simulink model "PEMFuelCellSystemWithACustomLibrary"  (R2025b)
settings: Solver=VariableStepAuto  StartTime=0.0  StopTime=2500  RelTol=1e-3  AbsTol=1e-3
model workspace: external: MATLAB File PEMFuelCellSystemWithACustomLibraryParameters.m (data not in the file)
values from neighbouring files (symbols this model uses):
  anode_tube_D = 0.01    [PEMFuelCellSystemWithACustomLibraryParameters.m]
  cathode_tube_D = 0.05    [PEMFuelCellSystemWithACustomLibraryParameters.m]
  comp_rpm_TLU = [0, 1800, 3600]    [PEMFuelCellSystemWithACustomLibraryParameters.m]
  coolant_num_layers = 20    [PEMFuelCellSystemWithACustomLibraryParameters.m]
  coolant_num_passes = 12    [PEMFuelCellSystemWithACustomLibraryParameters.m]
  coolant_tube_D = 0.05    [PEMFuelCellSystemWithACustomLibraryParameters.m]
  coolant_w_channels = 1    [PEMFuelCellSystemWithACustomLibraryParameters.m]
  env_p = 0.101325    [PEMFuelCellSystemWithACustomLibraryParameters.m]
  env_T = 20    [PEMFuelCellSystemWithACustomLibraryParameters.m]
  env_yH20 = env_RH * env_pSat_H2O / env_p    [PEMFuelCellSystemWithACustomLibraryParameters.m]
  env_yO2 = 0.21    [PEMFuelCellSystemWithACustomLibraryParameters.m]
  radiator_air_area_fins = 2 * radiator_N_fins * radiator_W * radiator_gap_H    (= 11.5625)    [PEMFuelCellSystemWithACustomLibraryParameters.m]
  radiator_air_area_primary = 2 * (radiator_N_tubes - 1) * radiator_W * (radiator_L + radiator_gap_H)    (= 1.223125)    [PEMFuelCellSystemWithACustomLibraryParameters.m]
  radiator_eta_fin = 0.7    [PEMFuelCellSystemWithACustomLibraryParameters.m]
  radiator_N_tubes = 25    [PEMFuelCellSystemWithACustomLibraryParameters.m]
  radiator_rho = 2700    [PEMFuelCellSystemWithACustomLibraryParameters.m]
  radiator_t_wall = 1e-4    (= 0.0001)    [PEMFuelCellSystemWithACustomLibraryParameters.m]
  radiator_tube_H = 0.0015    [PEMFuelCellSystemWithACustomLibraryParameters.m]
  radiator_W = 0.025    [PEMFuelCellSystemWithACustomLibraryParameters.m]
  stack_area = 280    [PEMFuelCellSystemWithACustomLibraryParameters.m]
  stack_iL = 1.4    [PEMFuelCellSystemWithACustomLibraryParameters.m]
  stack_mea_rho = 1800    [PEMFuelCellSystemWithACustomLibraryParameters.m]
  stack_num_cells = 400    [PEMFuelCellSystemWithACustomLibraryParameters.m]
  stack_num_channels = 8    [PEMFuelCellSystemWithACustomLibraryParameters.m]
  stack_t_gdl = 250    [PEMFuelCellSystemWithACustomLibraryParameters.m]
  stack_t_membrane = 125    [PEMFuelCellSystemWithACustomLibraryParameters.m]
  stack_w_channels = 1    [PEMFuelCellSystemWithACustomLibraryParameters.m]
libraries: fl_lib x57, FuelCell_lib x32, nesl_utility x24, slpidlib x2, simulink x1
(part 1 of 3)
CloseFcn:
  | try,close(h1_PEMFuelCellSystemWithACustomLibrary),end
  | clear h1_PEMFuelCellSystemWithACustomLibrary
  | try,close(h2_PEMFuelCellSystemWithACustomLibrary),end
  | clear h2_PEMFuelCellSystemWithACustomLibrary
  | try,close(h3_PEMFuelCellSystemWithACustomLibrary),end
  | clear h3_PEMFuelCellSystemWithACustomLibrary
  | try,close(h4_PEMFuelCellSystemWithACustomLibrary),end
  | clear h4_PEMFuelCellSystemWithACustomLibrary
  | try,close(h5_PEMFuelCellSystemWithACustomLibrary),end
  | clear h5_PEMFuelCellSystemWithACustomLibrary
  | try,close(h6_PEMFuelCellSystemWithACustomLibrary),end
  | clear h6_PEMFuelCellSystemWithACustomLibrary
  | 
  | clear tout simlog_PEMFuelCellSystemWithACustomLibrary
Description:
  | PEM Fuel Cell System with a Custom Library
settings Model: Creator=The MathWorks, Inc.  LastModifiedBy=The MathWorks, Inc.
settings SolverCC: AutoScaleAbsTol=off  MaxConsecutiveMinStep=10  AlgebraicLoopSolver=TrustRegion  MaxZcPerStep=1.0
settings DataIOCC: SaveFormat=Array  ReturnWorkspaceOutputs=off
settings DebuggingCC: UnconnectedInputMsg=warning  UnconnectedOutputMsg=warning  UnconnectedLineMsg=warning  SymbolicDimsDataTypeCodeGenerationDiagnostic=none
settings ModelReferenceCC: EnableRefExpFcnMdlSchedulingChecks=on
settings SFSimCC: CustomCodeUndefinedFunction=UseInterfaceOnly
settings RTWCC: GPUComputeCapability=3.5  DLArmComputeVersion=19.05
settings SimscapeCC: SimscapeLogType=all  SimscapeLogSimulationStatistics=on  SimscapeLogName=simlog_PEMFuelCellSystemWithACustomLibrary  SimscapeLogDataHistory=20000.0

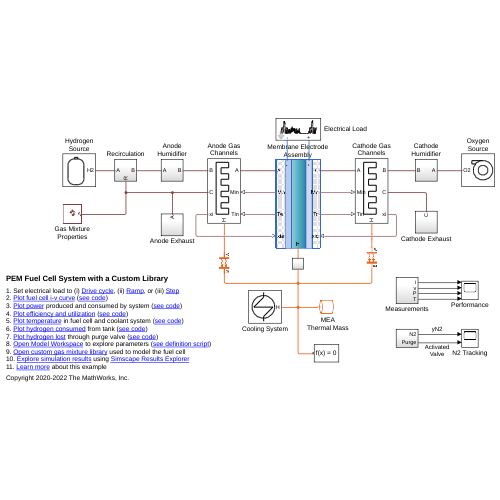
[thumbnail: Simulink's stored preview of the top-level diagram]
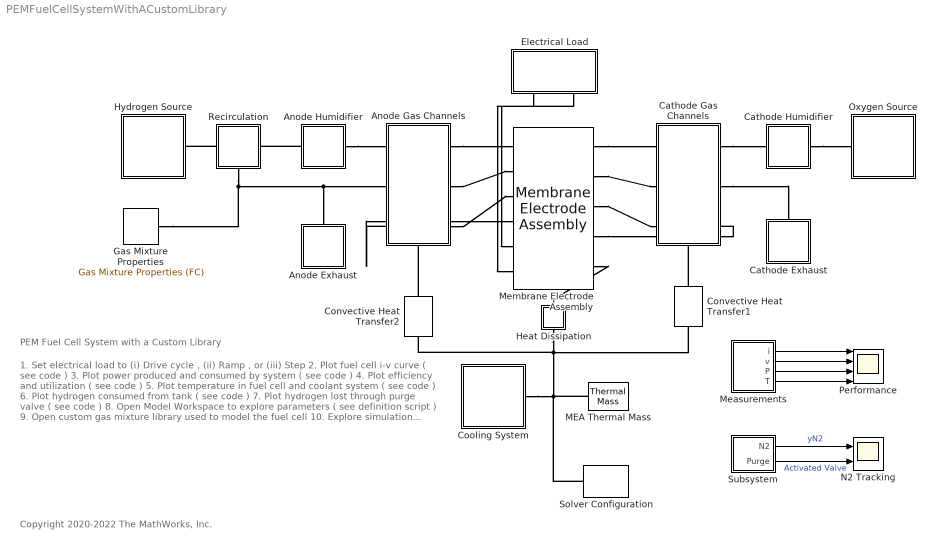
== system PEMFuelCellSystemWithACustomLibrary ==
  note: PEM Fuel Cell System with a Custom Library
  note: 1. Set electrical load to (i) Drive cycle , (ii) Ramp , or (iii) Step
      | 2. Plot fuel cell i-v curve ( see code )
      | 3. Plot power produced and consumed by system ( see code )
      | 4. Plot efficiency and utilization ( see code )
      | 5. Plot temperature in fuel cell and coolant system ( see code )
      | 6. Plot hydrogen consumed from tank ( see code )
      | 7. Plot hydrogen lost through purge valve ( see code )
      | 8. Open Model Workspace to explore parameters ( see definition script )
      | 9. Open custom gas mixture library used to model the fuel cell
      | 10. Explore simulation results using Simscape Results Explorer
      | 11. Learn more about this example
  note: Copyright 2020-2022 The MathWorks, Inc.
  Anode Humidifier : Subsystem  Tag=PublishSubsystem
  Anode Exhaust : Subsystem  Tag=PublishSubsystem
      settings: PortSchema="{\"entries\":[{\"content\":{\"sides\":[{\"content\":{\"connectorIds\":[]},\"type\":\"ConnectorPlacement.EquallySpacedRectSide\",\"uuid\":\"6344d1cf-22ea-4a51-9588-07afca0fac15\"},{\"content\":{\"connectorIds\":[],\"side\":\"RIGHT\"},\"type\":\"ConnectorPlacement.EquallySpacedRectSide\",\"uuid\":\"a3908f81-9410-4056-87cd-9faba76d3fb8\"},{\"content\":{\"connectorIds\":[\"LConn1\"],\"side\":\"TOP\"},\"type\":\"ConnectorPlacement.EquallySpacedRectSide\",\"uuid\":\"a1c9e24d-adb9-4361-8e9b-feafccbbdb81\"}]},\"type\":\"ConnectorPlacement.EquallySpacedConnector\",\"uuid\":\"d5180d8f-18a0-491d-9fff-909db43c9aea\"}],\"packageUris\":[\"http://schema.mathworks.com/mf0/Connector/R2020b\"],\"version\":\"1.0\"}"
  Anode Gas Channels : Subsystem  Tag=PublishSubsystem
      settings: PortSchema="{\"entries\":[{\"content\":{\"sides\":[{\"content\":{\"connectorIds\":[\"LConn1\",\"LConn2\",\"LConn3\"]},\"type\":\"ConnectorPlacement.EquallySpacedRectSide\",\"uuid\":\"f0c92738-2de1-40ac-9e4a-670524600aa2\"},{\"content\":{\"connectorIds\":[\"RConn1\",\"RConn2\",\"RConn3\"],\"side\":\"RIGHT\"},\"type\":\"ConnectorPlacement.EquallySpacedRectSide\",\"uuid\":\"f0ed995d-2dce-4bd6-9faa-b1cb502a30b1\"},{\"content\":{\"connectorIds\":[],\"side\":\"TOP\"},\"type\":\"ConnectorPlacement.EquallySpacedRectSide\",\"uuid\":\"b5d2d698-46b6-42b5-a767-bb9f1790aa28\"},{\"content\":{\"connectorIds\":[\"RConn4\"],\"side\":\"BOTTOM\"},\"type\":\"ConnectorPlacement.EquallySpacedRectSide\",\"uuid\":\"3e8c99a3-0044-43a9-bacb-b652445e4ac6\"}]},\"type\":\"ConnectorPlacement.EquallySpacedConnector\",\"uuid\":\"912925fb-ca80-4fe6-8a1d-a2308cfd6f88\"}],\"packageUris\":[\"http://schema.mathworks.com/mf0/Connector/R2020b\"],\"version\":\"1.0\"}"
      mask Display:
      | plot(0, 0)
      | plot(100, 100)
      | 
      | x1 = 25;
      | x2 = 65;
      | y1 = 23;
      | y2 = 95;
      | xt = 15;
      | yt = 9;
      | 
      | x_pattern = [x2 x2    x1+xt x1+xt   x1+xt   x2     ];
      | y_pattern = [y2 y2-yt y2-yt y2-2*yt y2-2*yt y2-2*yt];
      | 
      | plot([x1 x1 x2 x_pattern x_pattern      x_pattern      x_pattern         x2    x1], ...
      |      [y1-yt y2 y2 y_pattern y_pattern-2*yt y_pattern-4*yt y_pattern-6*yt y1-yt y1-yt])
  Cathode Humidifier : Subsystem  Tag=PublishSubsystem
  Cathode Exhaust : Subsystem  Tag=PublishSubsystem
      settings: PortSchema="{\"entries\":[{\"content\":{\"sides\":[{\"content\":{\"connectorIds\":[]},\"type\":\"ConnectorPlacement.EquallySpacedRectSide\",\"uuid\":\"6344d1cf-22ea-4a51-9588-07afca0fac15\"},{\"content\":{\"connectorIds\":[],\"side\":\"RIGHT\"},\"type\":\"ConnectorPlacement.EquallySpacedRectSide\",\"uuid\":\"a3908f81-9410-4056-87cd-9faba76d3fb8\"},{\"content\":{\"connectorIds\":[\"LConn1\"],\"side\":\"TOP\"},\"type\":\"ConnectorPlacement.EquallySpacedRectSide\",\"uuid\":\"a1c9e24d-adb9-4361-8e9b-feafccbbdb81\"}]},\"type\":\"ConnectorPlacement.EquallySpacedConnector\",\"uuid\":\"d5180d8f-18a0-491d-9fff-909db43c9aea\"}],\"packageUris\":[\"http://schema.mathworks.com/mf0/Connector/R2020b\"],\"version\":\"1.0\"}"
  Cathode Gas Channels : Subsystem  Tag=PublishSubsystem
      settings: PortSchema="{\"entries\":[{\"content\":{\"sides\":[{\"content\":{\"connectorIds\":[\"LConn1\",\"LConn2\",\"LConn3\"]},\"type\":\"ConnectorPlacement.EquallySpacedRectSide\",\"uuid\":\"f0c92738-2de1-40ac-9e4a-670524600aa2\"},{\"content\":{\"connectorIds\":[\"RConn1\",\"RConn2\",\"RConn3\"],\"side\":\"RIGHT\"},\"type\":\"ConnectorPlacement.EquallySpacedRectSide\",\"uuid\":\"f0ed995d-2dce-4bd6-9faa-b1cb502a30b1\"},{\"content\":{\"connectorIds\":[],\"side\":\"TOP\"},\"type\":\"ConnectorPlacement.EquallySpacedRectSide\",\"uuid\":\"b5d2d698-46b6-42b5-a767-bb9f1790aa28\"},{\"content\":{\"connectorIds\":[\"RConn4\"],\"side\":\"BOTTOM\"},\"type\":\"ConnectorPlacement.EquallySpacedRectSide\",\"uuid\":\"3e8c99a3-0044-43a9-bacb-b652445e4ac6\"}]},\"type\":\"ConnectorPlacement.EquallySpacedConnector\",\"uuid\":\"912925fb-ca80-4fe6-8a1d-a2308cfd6f88\"}],\"packageUris\":[\"http://schema.mathworks.com/mf0/Connector/R2020b\"],\"version\":\"1.0\"}"
      mask Display:
      | plot(0, 0)
      | plot(100, 100)
      | 
      | x1 = 25;
      | x2 = 65;
      | y1 = 23;
      | y2 = 95;
      | xt = 15;
      | yt = 9;
      | 
      | x_pattern = [x2 x2    x1+xt x1+xt   x1+xt   x2     ];
      | y_pattern = [y2 y2-yt y2-yt y2-2*yt y2-2*yt y2-2*yt];
      | 
      | plot([x1 x1 x2 x_pattern x_pattern      x_pattern      x_pattern         x2    x1], ...
      |      [y1-yt y2 y2 y_pattern y_pattern-2*yt y_pattern-4*yt y_pattern-6*yt y1-yt y1-yt])
  Convective Heat Transfer1 : fl_lib/Thermal/Thermal Elements/Convective Heat Transfer  thermal_type=foundation.enum.constant_variable.constant  area=stack_w_channels^2 * stack_num_channels * stack_num_cells cm^2  heat_tr_coeff=10 W/(m^2 * K)  min_heat_tr_coeff=1e-3 W/(K*m^2)  T_specify=off  T_priority=None  T=0 K  T_nominal_specify=off  T_nominal_value=1  T_nominal_unit=K  Q_specify=off  Q_priority=None  Q=0 W  Q_nominal_specify=off  Q_nominal_value=1  Q_nominal_unit=W
  Convective Heat Transfer2 : fl_lib/Thermal/Thermal Elements/Convective Heat Transfer  thermal_type=foundation.enum.constant_variable.constant  area=stack_w_channels^2 * stack_num_channels * stack_num_cells cm^2  heat_tr_coeff=10 W/(m^2 * K)  min_heat_tr_coeff=1e-3 W/(K*m^2)  T_specify=off  T_priority=None  T=0 K  T_nominal_specify=off  T_nominal_value=1  T_nominal_unit=K  Q_specify=off  Q_priority=None  Q=0 W  Q_nominal_specify=off  Q_nominal_value=1  Q_nominal_unit=W
  Cooling System : Subsystem  Tag=PublishSubsystem
      mask Display:
      | plot(0, 0)
      | plot(100, 100)
      | 
      | n = 80;
      | r = 35;
      | 
      | x = 45;
      | y = 50;
      | t = 5;
      | 
      | plot(cos(linspace(0, 2*pi, n))*r + x, sin(linspace(0, 2*pi, n))*r + y)
      | 
      | plot([x x x-r+t x+r-t x x], [y+r+2*t y+r-t y y y-r+t y-r-2*t])
  Electrical Load : Subsystem  Tag=PublishSubsystem  mask(Electrical Load){input_type=Drive cycle}
      mask prompts: input_type "Select one of the following scenarios:"
      settings: PortSchema="{\"entries\":[{\"content\":{\"sides\":[{\"content\":{\"connectorIds\":[]},\"type\":\"ConnectorPlacement.EquallySpacedRectSide\",\"uuid\":\"cf26c57a-4aaa-4eca-a1cf-dab3379228b7\"},{\"content\":{\"connectorIds\":[],\"side\":\"RIGHT\"},\"type\":\"ConnectorPlacement.EquallySpacedRectSide\",\"uuid\":\"bd4a28c6-f8d3-4492-9f61-a12eb17ccdd3\"},{\"content\":{\"connectorIds\":[],\"side\":\"TOP\"},\"type\":\"ConnectorPlacement.EquallySpacedRectSide\",\"uuid\":\"7f54a4db-ccf4-4e3a-a135-4ada067d241f\"},{\"content\":{\"connectorIds\":[\"RConn1\",\"RConn2\"],\"side\":\"BOTTOM\"},\"type\":\"ConnectorPlacement.EquallySpacedRectSide\",\"uuid\":\"8817983d-3f79-43b3-9594-6d12f7dcf066\"}]},\"type\":\"ConnectorPlacement.EquallySpacedConnector\",\"uuid\":\"79253ea6-cd7f-4983-840a-f5cee3a4dd91\"}],\"packageUris\":[\"http://schema.mathworks.com/mf0/Connector/R2020b\"],\"version\":\"1.0\"}"
      mask TypeOptions input_type: Drive cycle | Ramp | Step
      mask Callback input_type:
      | activeVariant = get_param(gcb, 'input_type');
      | set_param([gcb '/Inputs'], 'OverrideUsingVariant', activeVariant)
      mask Display:
      | blk = get_param([gcb, '/Inputs'], 'CompiledActiveChoiceBlock');
      | eval(get_param(blk, 'MaskDisplay'))
  Gas Mixture Properties : FuelCell_lib/utilities/Gas Mixture Properties (FC)  M=[.02801348; .0319988; .00201588; .018015268] kg/mol  T_LUT=[223.15, 228.15, 233.15, 238.15, 243.15, 248.15, 253.15, 258.15, 263.15, 268.15, 272.66, 273.15, 273.66, 278.15, 283.15, 288.15, 293.15, 298.15, 303.15, 308.15, 313.15, 318.15, 323.15, 328.15, 333.15, 338.15, 343.15, 348.15, 353.15, 358.15, 363.15, 368.15, 373.15, 378.15, 383.15, 388.15, 393.15, 398.15, 403.15, 408.15, 413.15, 418.15, 423.15, 428.15, 433.15, 438.15, 443.15, 448.15, 453.15, 458.15, 463.15, 468.15, 473.15, 478.15, 483.15, 488.15, 493.15, 498.15, 503.15, 508.15, 513.15, 518.15, 523.15, 528.15, 533.15, 538.15, 543.15, 548.15, 553.15, 558.15, 563.15, 568.15, 573.15, 578.15, 583.15, 588.15, 593.15, 598.15, 603.15, 608.15, 613.15, 618.15, 623.15, 628.15, 633.15, 638.15, 643.15, 646.596, 647.596, 648.15, 653.15, 658.15, 663.15, 668.15, 673.15, 678.15, 683.15, 688.15, 693.15, 698.15, 703.15, 708.15, 713.15, 718.15, 723.15, 728.15, 733.15, 738.15, 743.15, 748.15, 753.15, 758.15, 763.15, 768.15, 773.15] K  h=[231141.016491446, 236352.965205416, 241564.116942502, 246774.547965521, 251984.329578037, 257193.529102445, 262402.210743391, 267610.436352497, 272818.266107137, 278025.759113494, 282722.677545767, 283232.973942118, 283764.096522684, 288439.969102709, 293646.803463634, 298853.536620762, 304060.229219521, 309266.943233533, 314473.742202799, 319680.691434074, 324887.8581659, 330095.311700555, 335303.123505103, 340511.36728359, 345720.119022414, 350929.457010809, 356139.461838346, 361350.216371324, 366561.805709856, 371774.317127435, 376987.839994712, 382202.465689149, 387418.287492189, 392635.40047548, 397853.901377681, 403073.888473255, 408295.461434618, 413518.721188933, 418743.769770759, 423970.710171682, 429199.646187988, 434430.682267366, 439663.923355528, 444899.474743584, 450137.441916926, 455377.930406292, 460621.045641629, 465866.892809302, 471115.576713123, 476367.201639612, 481621.871227875, 486879.688344373, 492140.754962869, 497405.17204973, 502673.03945477, 507944.455807744, 513219.518420569, 518498.32319534, 523780.964538135, 529067.535278613, 534358.126595352, 539652.827946877, 544951.727008291, 550254.909613398, 555562.459702215, 560874.459273737, 566190.9883438, 571512.124907907, 576837.944908841, 582168.5222089, 587503.928566583, 592844.233617549, 598189.504859656, 603539.807641917, 608895.205157175, 614255.758438318, 619621.526357853, 624992.565630662, 630368.93081975, 635750.674344825, 641137.846493532, 646530.495435168, 651928.66723672, 657332.405881072, 662741.753287217, 668156.749332323, 673577.431875525, 677316.695180152, 678402.308157762, 679003.836783286, 684435.997956195, 689873.947357094, 695317.715040376, 700767.329182368, 706222.816112665, 711684.200346327, 717151.504616806, 722624.74990955, 728103.955496141, 733589.138968926, 739080.316276029, 744577.501756671, 750080.708176737, 755589.946764509, 761105.227246498, 766626.557883331, 772153.94550561, 777687.395549719, 783226.912093505, 788772.497891803, 794324.154411751, 799881.881867868, 805445.679256845, 811015.544392026, 816591.473937548; 202302.438243561, 206873.832702735, 211445.560194856, 216017.841858298, 220590.899229627, 225164.954671145, 229740.23159406, 234316.954511722, 238895.348953335, 243475.641264836, 247608.881176925, 248058.058320402, 248525.59321637, 252642.82716507, 257230.174606287, 261820.326769861, 266413.508633549, 271009.943549664, 275609.852766255, 280213.454954912, 284820.965751807, 289432.597317356, 294048.5579188, 298669.051538973, 303294.277513762, 307924.430199932, 312559.698674411, 317200.266465557, 321846.311316458, 326498.00497993, 331155.513044569, 335818.994790904, 340488.60307654, 345164.484248972, 349846.778084642, 354535.617752736, 359231.129802116, 363933.43416981, 368642.64420942, 373358.866737839, 378082.202098712, 382812.74424106, 387550.580811602, 392295.793259308, 397048.456950805, 401808.641295332, 406576.409877989, 411351.820600107, 416134.925825648, 420925.772532589, 425724.402468363, 430530.852308438, 435345.153817243, 440167.334010684, 444997.415319553, 449835.415753221, 454681.349063045, 459535.224904964, 464397.049000843, 469266.823298151, 474144.546127596, 479030.212358419, 483923.813551045, 488825.338106863, 493734.77141492, 498652.095995354, 503577.291639419, 508510.33554598, 513451.202454384, 518399.864773635, 523356.292707817, 528320.45437773, 533292.31593873, 538271.841694755, 543258.994208562, 548253.734408192, 553256.021689693, 558265.814016148, 563283.068013058, 568307.739060136, 573339.78137958, 578379.148120885, 583425.791442281, 588479.662588863, 593540.711967502, 598608.889218605, 603684.143284836, 607186.10084207, 608202.961489427, 608766.422476851, 613855.674536152, 618951.846695155, 624054.885734541, 629164.738037977, 634281.349644321, 639404.666297356, 644534.633493177, 649671.196525283, 654814.300527474, 659963.890514636, 665119.911421476, 670282.308139299, 675451.025550903, 680626.008563655, 685807.202140829, 690994.551331273, 696188.001297474, 701387.497342081, ...(+4242 chars)] J/kg  pSat=[3379.45709837364, 3379.45809837364, 3379.45909837364, 3379.46009837364, 3379.46109837364, 3379.46209837364, 3379.46309837364, 3379.46409837364, 3379.46509837364, 3379.46609837364, 3379.46709837364, 3379.46809837364, 3379.46909837364, 3379.47009837364, 3379.47109837364, 3379.47209837364, 3379.47309837364, 3379.47409837364, 3379.47509837364, 3379.47609837364, 3379.47709837364, 3379.47809837364, 3379.47909837364, 3379.48009837364, 3379.48109837364, 3379.48209837364, 3379.48309837364, 3379.48409837364, 3379.48509837364, 3379.48609837364, 3379.48709837364, 3379.48809837364, 3379.48909837364, 3379.49009837364, 3379.49109837364, 3379.49209837364, 3379.49309837364, 3379.49409837364, 3379.49509837364, 3379.49609837364, 3379.49709837364, 3379.49809837364, 3379.49909837364, 3379.50009837364, 3379.50109837364, 3379.50209837364, 3379.50309837364, 3379.50409837364, 3379.50509837364, 3379.50609837364, 3379.50709837364, 3379.50809837364, 3379.50909837364, 3379.51009837364, 3379.51109837364, 3379.51209837364, 3379.51309837364, 3379.51409837364, 3379.51509837364, 3379.51609837364, 3379.51709837364, 3379.51809837364, 3379.51909837364, 3379.52009837364, 3379.52109837364, 3379.52209837364, 3379.52309837364, 3379.52409837364, 3379.52509837364, 3379.52609837364, 3379.52709837364, 3379.52809837364, 3379.52909837364, 3379.53009837364, 3379.53109837364, 3379.53209837364, 3379.53309837364, 3379.53409837364, 3379.53509837364, 3379.53609837364, 3379.53709837364, 3379.53809837364, 3379.53909837364, 3379.54009837364, 3379.54109837364, 3379.54209837364, 3379.54309837364, 3379.54409837364, 3379.54509837364, 3379.54609837364, 3379.54709837364, 3379.54809837364, 3379.54909837364, 3379.55009837364, 3379.55109837364, 3379.55209837364, 3379.55309837364, 3379.55409837364, 3379.55509837364, 3379.55609837364, 3379.55709837364, 3379.55809837364, 3379.55909837364, 3379.56009837364, 3379.56109837364, 3379.56209837364, 3379.56309837364, 3379.56409837364, 3379.56509837364, 3379.56609837364, 3379.56709837364, 3379.56809837364, 3379.56909837364, 3379.57009837364, 3379.57109837364; 5023.40410987222, 5023.40510987222, 5023.40610987222, 5023.40710987222, 5023.40810987222, 5023.40910987222, 5023.41010987222, 5023.41110987222, 5023.41210987222, 5023.41310987222, 5023.41410987222, 5023.41510987222, 5023.41610987222, 5023.41710987222, 5023.41810987222, 5023.41910987222, 5023.42010987222, 5023.42110987222, 5023.42210987222, 5023.42310987222, 5023.42410987222, 5023.42510987222, 5023.42610987222, 5023.42710987222, 5023.42810987222, 5023.42910987222, 5023.43010987222, 5023.43110987222, 5023.43210987222, 5023.43310987222, 5023.43410987222, 5023.43510987222, 5023.43610987222, 5023.43710987222, 5023.43810987222, 5023.43910987222, 5023.44010987222, 5023.44110987222, 5023.44210987222, 5023.44310987222, 5023.44410987222, 5023.44510987222, 5023.44610987222, 5023.44710987222, 5023.44810987222, 5023.44910987222, 5023.45010987222, 5023.45110987222, 5023.45210987222, 5023.45310987222, 5023.45410987222, 5023.45510987222, 5023.45610987222, 5023.45710987222, 5023.45810987222, 5023.45910987222, 5023.46010987222, 5023.46110987222, 5023.46210987222, 5023.46310987222, 5023.46410987222, 5023.46510987222, 5023.46610987222, 5023.46710987222, 5023.46810987222, 5023.46910987222, 5023.47010987222, 5023.47110987222, 5023.47210987222, 5023.47310987222, 5023.47410987222, 5023.47510987222, 5023.47610987222, 5023.47710987222, 5023.47810987222, 5023.47910987222, 5023.48010987222, 5023.48110987222, 5023.48210987222, 5023.48310987222, 5023.48410987222, 5023.48510987222, 5023.48610987222, 5023.48710987222, 5023.48810987222, 5023.48910987222, 5023.49010987222, 5023.49110987222, 5023.49210987222, 5023.49310987222, 5023.49410987222, 5023.49510987222, 5023.49610987222, 5023.49710987222, 5023.49810987222, 5023.49910987222, 5023.50010987222, 5023.50110987222, 5023.50210987222, 5023.50310987222, 5023.50410987222, 5023.50510987222, 5023.50610987222, 5023.50710987222, 5023.50810987222, 5023.50910987222, 5023.51010987222, ...(+4285 chars)] kPa  hfg=[1e-06, 1e-06, 1e-06, 1e-06, 1e-06, 1e-06, 1e-06, 1e-06, 1e-06, 1e-06, 1e-06, 1e-06, 1e-06, 1e-06, 1e-06, 1e-06, 1e-06, 1e-06, 1e-06, 1e-06, 1e-06, 1e-06, 1e-06, 1e-06, 1e-06, 1e-06, 1e-06, 1e-06, 1e-06, 1e-06, 1e-06, 1e-06, 1e-06, 1e-06, 1e-06, 1e-06, 1e-06, 1e-06, 1e-06, 1e-06, 1e-06, 1e-06, 1e-06, 1e-06, 1e-06, 1e-06, 1e-06, 1e-06, 1e-06, 1e-06, 1e-06, 1e-06, 1e-06, 1e-06, 1e-06, 1e-06, 1e-06, 1e-06, 1e-06, 1e-06, 1e-06, 1e-06, 1e-06, 1e-06, 1e-06, 1e-06, 1e-06, 1e-06, 1e-06, 1e-06, 1e-06, 1e-06, 1e-06, 1e-06, 1e-06, 1e-06, 1e-06, 1e-06, 1e-06, 1e-06, 1e-06, 1e-06, 1e-06, 1e-06, 1e-06, 1e-06, 1e-06, 1e-06, 1e-06, 1e-06, 1e-06, 1e-06, 1e-06, 1e-06, 1e-06, 1e-06, 1e-06, 1e-06, 1e-06, 1e-06, 1e-06, 1e-06, 1e-06, 1e-06, 1e-06, 1e-06, 1e-06, 1e-06, 1e-06, 1e-06, 1e-06, 1e-06, 1e-06, 1e-06, 1e-06; 1e-06, 1e-06, 1e-06, 1e-06, 1e-06, 1e-06, 1e-06, 1e-06, 1e-06, 1e-06, 1e-06, 1e-06, 1e-06, 1e-06, 1e-06, 1e-06, 1e-06, 1e-06, 1e-06, 1e-06, 1e-06, 1e-06, 1e-06, 1e-06, 1e-06, 1e-06, 1e-06, 1e-06, 1e-06, 1e-06, 1e-06, 1e-06, 1e-06, 1e-06, 1e-06, 1e-06, 1e-06, 1e-06, 1e-06, 1e-06, 1e-06, 1e-06, 1e-06, 1e-06, 1e-06, 1e-06, 1e-06, 1e-06, 1e-06, 1e-06, 1e-06, 1e-06, 1e-06, 1e-06, 1e-06, 1e-06, 1e-06, 1e-06, 1e-06, 1e-06, 1e-06, 1e-06, 1e-06, 1e-06, 1e-06, 1e-06, 1e-06, 1e-06, 1e-06, 1e-06, 1e-06, 1e-06, 1e-06, 1e-06, 1e-06, 1e-06, 1e-06, 1e-06, 1e-06, 1e-06, 1e-06, 1e-06, 1e-06, 1e-06, 1e-06, 1e-06, 1e-06, 1e-06, 1e-06, 1e-06, 1e-06, 1e-06, 1e-06, 1e-06, 1e-06, 1e-06, 1e-06, 1e-06, 1e-06, 1e-06, 1e-06, 1e-06, 1e-06, 1e-06, 1e-06, 1e-06, 1e-06, 1e-06, 1e-06, 1e-06, 1e-06, 1e-06, 1e-06, 1e-06, 1e-06; 1e-06, 1e-06, 1e-06, 1e-06, 1e-06, 1e-06, 1e-06, 1e-06, 1e-06, 1e-06, 1e-06, 1e-06, 1e-06, 1e-06, 1e-06, 1e-06, 1e-06, 1e-06, 1e-06, 1e-06, 1e-06, 1e-06, 1e-06, 1e-06, 1e-06, 1e-06, 1e-06, 1e-06, 1e-06, 1e-06, 1e-06, 1e-06, 1e-06, 1e-06, 1e-06, 1e-06, 1e-06, 1e-06, 1e-06, 1e-06, 1e-06, 1e-06, 1e-06, 1e-06, 1e-06, 1e-06, 1e-06, 1e-06, 1e-06, 1e-06, 1e-06, 1e-06, 1e-06, 1e-06, 1e-06, 1e-06, 1e-06, 1e-06, 1e-06, 1e-06, 1e-06, 1e-06, 1e-06, 1e-06, 1e-06, 1e-06, 1e-06, 1e-06, 1e-06, 1e-06, 1e-06, 1e-06, 1e-06, 1e-06, 1e-06, 1e-06, 1e-06, 1e-06, 1e-06, 1e-06, 1e-06, 1e-06, 1e-06, 1e-06, 1e-06, 1e-06, 1e-06, 1e-06, 1e-06, 1e-06, 1e-06, 1e-06, 1e-06, 1e-06, 1e-06, 1e-06, 1e-06, 1e-06, 1e-06, 1e-06, 1e-06, 1e-06, 1e-06, 1e-06, 1e-06, 1e-06, 1e-06, 1e-06, 1e-06, 1e-06, 1e-06, 1e-06, 1e-06, 1e-06, 1e-06; 2837864.08019577, 2838359.64755355, 2838666.81898809, 2838784.77034599, 2838713.54467034, 2838454.24787559, 2838009.25741655, 2837382.44395187, 2836579.40600181, 2835607.71760031, 2834594.67651108, 2834477.18894141, 2499722.30618946, 2489041.99020784, 2477187.06302236, 2465351.7416476, 2453519.25941972, 2441676.17491261, 2429811.22987555, 2417914.58528419, 2405977.2867868, 2393990.8796467, 2381947.12654054, 2369837.79867559, 2357654.52030374, 2345388.65272411, 2333031.20800926, 2320572.78571749, 2308003.52809268, 2295313.09085395, 2282490.62771799, 2269524.78734365, 2256403.72152658, 2243115.10329165, 2229646.15315164, 2215983.67133732, 2202114.07337171, 2188023.4260502, 2173697.4807639, 2159121.70119209, 2144281.28268552, 2129161.16112867, 2113746.00964951, 2098020.2221716, 2081967.88340889, 2065572.72542774, 2048818.07129851, 2031686.76660156, 2014161.09962583, 1996222.71100774, 1977852.4933118, 1959030.48067786, 1939735.72816654, 1919946.17983732, 1899638.52389864, 1878788.03248115, 1857368.38273035, 1835351.45503499, 1812707.10332357, 1789402.89139924, 1765403.7880462, 1740671.81185592, 1715165.61416478, 1688839.98508869, 1661645.26339623, 1633526.62581446, 1604423.22494339, 1574267.13647052, 1542982.06457038, 1510481.73749009, 1476667.90089116, 1441427.7808096, 1404630.83498412, 1366124.53003558, 1325728.75296441, 1283228.25127755, 1238362.12284385, 1190808.69353032, 1140162.81350073, 1085900.00650484, 1027316.58328831, 963423.535757087, 892746.804215804, 812925.386717866, 719827.862875472, 605175.851189099, 443831.042740307, 207325.498642852, 1e-06, 1e-06, 1e-06, 1e-06, 1e-06, 1e-06, 1e-06, 1e-06, 1e-06, 1e-06, 1e-06, 1e-06, 1e-06, 1e-06, 1e-06, 1e-06, 1e-06, 1e-06, 1e-06, 1e-06, 1e-06, 1e-06, 1e-06, 1e-06, 1e-06, 1e-06, 1e-06] J/kg  visc=[1.41367187227787e-05, 1.43951114487243e-05, 1.46513505943947e-05, 1.49054792333128e-05, 1.51575394313155e-05, 1.54075722530882e-05, 1.56556177723748e-05, 1.59017150851275e-05, 1.61459023249833e-05, 1.63882166805598e-05, 1.66052077736712e-05, 1.66286944141481e-05, 1.6653121321316e-05, 1.68673708814506e-05, 1.71042805520748e-05, 1.73394570305386e-05, 1.75729330775902e-05, 1.78047406316744e-05, 1.80349108304122e-05, 1.82634740319801e-05, 1.84904598362994e-05, 1.87158971059617e-05, 1.89398139868313e-05, 1.91622379282776e-05, 1.93831957030016e-05, 1.96027134264274e-05, 1.98208165756394e-05, 2.00375300078486e-05, 2.02528779783805e-05, 2.0466884158177e-05, 2.06795716508121e-05, 2.08909630090209e-05, 2.11010802507466e-05, 2.13099448747091e-05, 2.15175778755041e-05, 2.17239997582382e-05, 2.19292305527123e-05, 2.21332898271596e-05, 2.23361967015518e-05, 2.25379698604828e-05, 2.27386275656414e-05, 2.29381876678842e-05, 2.3136667618921e-05, 2.33340844826236e-05, 2.3530454945969e-05, 2.37257953296299e-05, 2.39201215982222e-05, 2.41134493702215e-05, 2.43057939275585e-05, 2.44971702249056e-05, 2.46875928986634e-05, 2.48770762756575e-05, 2.50656343815568e-05, 2.5253280949021e-05, 2.54400294255878e-05, 2.56258929813084e-05, 2.58108845161405e-05, 2.59950166671062e-05, 2.61783018152239e-05, 2.63607520922219e-05, 2.65423793870414e-05, 2.67231953521356e-05, 2.6903211409573e-05, 2.7082438756951e-05, 2.72608883731268e-05, 2.74385710237722e-05, 2.76154972667571e-05, 2.77916774573698e-05, 2.79671217533781e-05, 2.8141840119937e-05, 2.83158423343493e-05, 2.84891379906823e-05, 2.86617365042478e-05, 2.88336471159483e-05, 2.90048788964945e-05, 2.91754407504992e-05, 2.93453414204507e-05, 2.95145894905704e-05, 2.96831933905586e-05, 2.98511613992321e-05, 3.00185016480563e-05, 3.01852221245778e-05, 3.03513306757577e-05, 3.05168350112115e-05, 3.06817427063567e-05, 3.08460612054727e-05, 3.10097978246753e-05, 3.11223101484351e-05, 3.11549095027834e-05, 3.11729597548076e-05, 3.13355540642517e-05, 3.14975877016632e-05, 3.16590674986295e-05, 3.18200001722572e-05, 3.1980392327688e-05, 3.21402504605474e-05, 3.22995809593273e-05, 3.24583901077048e-05, 3.26166840867995e-05, 3.27744689773707e-05, 3.29317507619573e-05, 3.30885353269602e-05, 3.32448284646722e-05, 3.34006358752535e-05, 3.35559631686569e-05, 3.37108158665036e-05, 3.386519940391e-05, 3.40191191312693e-05, 3.41725803159864e-05, 3.43255881441702e-05, 3.44781477222827e-05, 3.46302640787471e-05, 3.47819421655153e-05, 3.49331868595976e-05, 3.50840029645535e-05; 1.61727625939969e-05, 1.64800348163752e-05, 1.67849249289461e-05, 1.70874763385104e-05, 1.73877314906162e-05, 1.76857318827313e-05, 1.79815180787588e-05, 1.82751297246631e-05, 1.85666055649935e-05, 1.88559834601223e-05, 1.91152334141466e-05, 1.91433004040297e-05, 1.91724923335051e-05, 1.94285925424925e-05, 1.97118951915503e-05, 1.99932428561378e-05, 2.02726692487909e-05, 2.0550207308342e-05, 2.08258892185376e-05, 2.10997464265164e-05, 2.13718096610994e-05, 2.1642108950849e-05, 2.19106736418628e-05, 2.2177532415273e-05, 2.24427133044281e-05, 2.27062437117386e-05, 2.29681504251728e-05, 2.32284596343903e-05, 2.34871969465072e-05, 2.37443874014869e-05, 2.40000554871539e-05, 2.42542251538295e-05, 2.45069198285914e-05, 2.47581624291569e-05, 2.50079753773964e-05, 2.52563806124785e-05, 2.55033996036544e-05, 2.57490533626856e-05, 2.5993362455923e-05, 2.62363470160433e-05, 2.64780267534498e-05, 2.67184209673466e-05, 2.69575485564922e-05, 2.71954280296414e-05, 2.74320775156834e-05, 2.76675147734838e-05, 2.79017572014382e-05, 2.81348218467465e-05, 2.83667254144148e-05, 2.85974842759925e-05, 2.88271144780531e-05, 2.90556317504262e-05, 2.92830515141873e-05, 2.95093888894135e-05, 2.97346587027121e-05, 2.99588754945282e-05, 3.01820535262398e-05, 3.04042067870451e-05, 3.06253490006501e-05, 3.08454936317613e-05, 3.10646538923909e-05, 3.12828427479797e-05, 3.15000729233431e-05, 3.17163569084472e-05, 3.19317069640184e-05, 3.21461351269937e-05, 3.23596532158154e-05, ...(+6081 chars)] Pa*s  kth=[.0201533289598555, .0205498478977229, .0209436243479093, .021334709172853, .0217231523299053, .0221090026803599, .0224923062983423, .0228731194697501, .0232514823102791, .0236274403134218, .0239645285405068, .024001038025113, .0240390140639034, .0243723190468717, .0247413260420822, .0251081007448699, .0254726839711067, .0258351156311544, .0261954347440081, .0265536794525567, .0269098870397153, .027264093945225, .0276163357829442, .0279666473584816, .0283150626870459, .0286616150114057, .0290063368198683, .0293492598642035, .0296904151774483, .0300298330915396, .030367543254732, .0307035746487643, .0310379556057464, .0313707138247415, .0317018763880283, .0320314697770248, .0323595198878675, .0326860520466354, .0330110910242146, .0333346610508026, .0336567858300489, .0339774885528352, .0342967919106956, .034614718108882, .034931288879077, .0352465254917613, .0355604487682404, .0358730790923364, .0361844364217532, .0364945402991202, .0368034098627232, .0371110638569293, .0374175206423128, .0377227982054912, .0380269141686771, .0383298857989552, .0386317300172905, .038932463407277, .039232102223632, .0395306624004454, .0398281595591903, .0401246090165013, .0404200257917289, .0407144246142751, .0410078199307183, .041300225911733, .0415916564588103, .041882125210787, .0421716455501863, .0424602306093797, .0427478932765718, .0430346462016167, .0433205018016684, .0436054722666738, .0438895695647092, .0441728054471687, .0444551914538068, .0447367389176411, .0450174589697189, .0452973625437518, .0455764603806227, .0458547630327692, .0461322808684469, .0464090240758773, .0466850026672817, .0469602264828077, .0472347051943485, .047423447165998, .0474781535175432, .047508448309261, .0477814651739835, .048053764977558, .0483253567550585, .0485962493909293, .0488664516222353, .0491359720418269, .0494048191014234, .049673001114615, .0499405262597882, .0502074025829757, .0504736380006326, .0507392403023426, .0510042171534549, .0512685760976542, .0515323245594664, .051795469846701, .0520580191528325, .0523199795593227, .0525813580378852, .0528421614526945, .0531023965625398, .0533620700229272, .05362118838813, .0538797581131894, .054137785555867; .020222476497919, .0206445807022053, .0210645207571161, .0214823269702069, .0218980296802622, .0223116591743438, .0227232456175504, .0231328189936544, .0235404090550529, .0239460452806985, .0243102773636833, .02434975684085, .0243908283884428, .0247515725676043, .0251515209302184, .0255496300141004, .0259459275017263, .0263404406510994, .0267331962526519, .0271242203353896, .0275135401488042, .0279011817294094, .0282871691008179, .0286715269894326, .0290542796887646, .0294354510617025, .0298150645436306, .0301931431462672, .0305697094621136, .0309447856694174, .0313183935375638, .0316905544328228, .0320612893243854, .0324306187906343, .0327985630255983, .033165141845547, .0335303746956895, .0338942806569427, .0342568784527416, .0346181864558669, .034978222695267, .0353370048628582, .0356945503202846, .0360508761056257, .0364059989400391, .0367599352343282, .0371127010954278, .0374643123327981, .0378147844647235, .0381641327245104, .0385123720665796, .0388595171724516, .0392055824566211, .0395505820723193, .039894529917164, .0402374396386945, .0405793246397936, .0409201980839948, .041260072900676, .0415989617901403, .041936877228585, .0422738314729596, .0426098365657135, .0429449043394367, .0432790464213934, .0436122742379499, .0439445990189012, .044276031801694, .0446065834355525, .0449362645855046, .0452650857363144, .0455930571963195, .0459201891011779, .0462464914175248, .0465719739465414, .0468966463274387, .0472205180408575, .0475435984121861, .0478658966147994, .0481874216732185, .048508182466196, .0488281877297258, .0491474460599816, .0494659659161843, .0497837556234006, .0501008233752753, .0504171772366974, .050634796910971, .0506978858908842, .050732825146403, .0510477749195164, .0513620342500299, .0516756107132256, .0519885117680394, .0523007447593693, .0526123169203288, .0529232353744476, ...(+4563 chars)] W/(K*m)  cp=[1042.47481613525, 1042.30740972221, 1042.15582350855, 1042.01895923372, 1041.89592698189, 1041.7860203931, 1041.68869544829, 1041.60355210019, 1041.5303181801, 1041.46883513431, 1041.42340759174, 1041.41904524216, 1041.41462436426, 1041.38098004563, 1041.35474978158, 1041.34053365648, 1041.33857084161, 1041.34915209664, 1041.37261195264, 1041.40932140332, 1041.4596810669, 1041.52411479091, 1041.60306367947, 1041.69698052785, 1041.80632465214, 1041.93155710441, 1042.07313626442, 1042.23151379957, 1042.40713098442, 1042.60041537083, 1042.81177779883, 1043.0416097375, 1043.29028094454, 1043.55813743188, 1043.84549972427, 1044.15266139706, 1044.4798878784, 1044.82741550134, 1045.19545079027, 1045.58416996649, 1045.99371865733, 1046.42421179343, 1046.87573367901, 1047.34833821997, 1047.84204929545, 1048.35686125845, 1048.89273955192, 1049.44962142723, 1050.02741675231, 1050.62600889779, 1051.24525568957, 1051.88499041755, 1052.54502289024, 1053.22514052633, 1053.92510947429, 1054.64467575236, 1055.38356640143, 1056.14149064423, 1056.91814104472, 1057.71319466223, 1058.52631419534, 1059.35714911116, 1060.20533675608, 1061.07050344451, 1061.95226552262, 1062.85023040452, 1063.76399757869, 1064.69315958273, 1065.63730294499, 1066.5960090919, 1067.56885521995, 1068.55541513176, 1069.55526003578, 1070.56795930928, 1071.5930812248, 1072.63019363995, 1073.678864651, 1074.73866321067, 1075.80915971051, 1076.8899265287, 1077.98053854387, 1079.08057361577, 1080.18961303367, 1081.3072419334, 1082.43304968401, 1083.56663024501, 1084.7075824953, 1085.49801103619, 1085.72798862852, 1085.85551053475, 1087.01002395946, 1088.17073811197, 1089.33727430716, 1090.50926003523, 1091.68632914257, 1092.8681219917, 1094.05428560121, 1095.24447376682, 1096.43834716441, 1097.63557343613, 1098.83582726038, 1100.03879040669, 1101.24415177639, 1102.45160742974, 1103.6608606007, 1104.87162169972, 1106.08360830573, 1107.29654514771, 1108.51016407688, 1109.7242040299, 1110.93841098393, 1112.15253790416, 1113.36634468425, 1114.57959808048, 1115.79207163994; 914.260336201333, 914.304824668748, 914.393541243093, 914.526507279298, 914.703852601414, 914.925770883161, 915.19248236135, 915.504203018565, 915.861119462566, 916.263368810086, 916.665145556483, 916.711022953181, 916.759236043945, 917.204076648534, 917.742438925491, 918.325927358406, 918.954264793829, 919.627078164243, 920.343899057692, 921.104165747365, 921.907226417208, 922.75234334921, 923.638697865235, 924.565395841369, 925.531473635794, 926.535904292228, 927.577603900203, 928.655438010848, 929.768228022569, 930.914757465176, 932.093778123631, 933.304015953838, 934.54417675283, 935.812951554468, 937.109021729373, 938.431063774449, 939.77775378303, 941.147771591598, 942.539804603054, 943.952551290037, 945.384724384585, 946.835053762746, 948.302289034591, 949.785201851517, 951.282587943779, 952.793268901984, 954.316093716732, 955.849940090922, 957.39371553924, 958.946358289353, 960.50683799903, 962.074156303174, 963.647347204262, 965.225477319277, 966.807645995638, 968.392985308112, 969.98065994805, 971.56986701573, 973.159835725945, 974.749827036359, 976.339133207575, 977.927077303213, 979.51301263777, 981.096322179429, 982.676417914447, 984.252740179265, 985.824756965931, 987.391963206008, 988.953880037653, 990.510054060155, 992.06005657981, 993.60348285064, 995.139951313124, 996.66910283376, 998.190599948012, 999.704126108867, 1001.20938494301, 1002.70609951638, 1004.19401161056, 1005.67288101144, 1007.14248481122, 1008.60261672466, 1010.05308642055, 1011.49371886888, 1012.92435370437, 1014.34484460677, 1015.75505869812, 1016.72093300515, 1017.00029181561, 1017.15487595739, 1018.54418865243, 1019.92290078942, 1021.29092757975, 1022.64819492427, 1023.99463891472, 1025.33020535231, 1026.65484928309, 1027.96853454986, 1029.27123336048, 1030.56292587207, 1031.84359979097, 1033.1132499879, 1034.37187812814, 1035.61949231623, 1036.85610675485, 1038.08174141746, 1039.29642173435, 1040.50017829166, ...(+4247 chars)] J/(K*kg)  s=[6533.45572452608, 6556.55416691419, 6579.14838843465, 6601.26011227968, 6622.90968678934, 6644.11620139082, 6664.89759051369, 6685.27072695501, 6705.25150595787, 6724.85492109068, 6742.22526410746, 6744.09513286678, 6746.03775547765, 6762.98553091904, 6781.53879043801, 6799.76692349242, 6817.6813257737, 6835.29281924035, 6852.61169108112, 6869.6477293672, 6886.41025572099, 6902.90815529234, 6919.14990430093, 6935.14359537533, 6950.89696089487, 6966.41739451858, 6981.71197106649, 6996.78746490169, 7011.65036694664, 7026.30690045397, 7040.76303564008, 7055.02450327961, 7069.09680734904, 7082.98523679979, 7096.69487653317, 7110.23061764303, 7123.5971669859, 7136.79905613283, 7149.84064975219, 7162.72615346843, 7175.45962123757, 7188.04496227668, 7200.48594758137, 7212.78621606213, 7224.94928032805, 7236.97853214348, 7248.87724758154, 7260.64859189598, 7272.29562413124, 7283.82130148882, 7295.22848346674, 7306.51993578718, 7317.69833412657, 7328.76626766078, 7339.72624243749, 7350.58068458659, 7361.33194337865, 7371.98229414078, 7382.5339410385, 7392.98901973147, 7403.34959991047, 7413.61768772242, 7423.79522808964, 7433.88410692935, 7443.8861532787, 7453.80314133043, 7463.63679238381, 7473.38877671533, 7483.06071537312, 7492.65418189894, 7502.17070398134, 7511.61176504332, 7520.97880576754, 7530.27322556212, 7539.49638396976, 7548.64960202269, 7557.73416354601, 7566.75131641163, 7575.70227374502, 7584.58821508682, 7593.41028751122, 7602.16960670301, 7610.8672579949, 7619.50429736692, 7628.08175240938, 7636.60062325083, 7645.06188345255, 7650.86034452878, 7652.53801393802, 7653.46648087081, 7661.81533848818, 7670.10935521525, 7678.34940666367, 7686.5363458919, 7694.67100412449, 7702.75419144608, 7710.78669747095, 7718.76929198912, 7726.70272558995, 7734.58773026386, 7742.42501998328, 7750.21529126338, 7757.95922370342, 7765.65748050945, 7773.31070899898, 7780.91954108838, 7788.48459376352, 7796.00646953438, 7803.48575687412, 7810.92303064324, 7818.31885249933, 7825.67377129291, 7832.98832344995, 7840.26303334147, 7847.49841364064; 6141.75750723404, 6162.01711770798, 6181.83895051213, 6201.24252376203, 6220.24614045623, 6238.86698916623, 6257.12123386815, 6275.02409432044, 6292.58991819632, 6309.83224600157, 6325.11795895991, 6326.76386966431, 6328.47391530252, 6343.39688556002, 6359.74274263025, 6375.81228616465, 6391.61579773949, 6407.16303174128, 6422.46324884818, 6437.52524679405, 6452.35738869901, 6466.96762921486, 6481.36353870324, 6495.55232563779, 6509.54085739918, 6523.33567961145, 6536.94303415158, 6550.3688759488, 6563.61888867747, 6576.69849943578, 6589.61289249305, 6602.3670221793, 6614.96562498355, 6627.41323092064, 6639.71417422029, 6651.87260338745, 6663.8924906779, 6675.77764102965, 6687.53170048661, 6699.15816414837, 6710.66038367655, 6722.04157438633, 6733.30482194886, 6744.45308872885, 6755.48921977945, 6766.41594851486, 6777.23590208011, 6787.95160643542, 6798.56549117191, 6809.07989407407, 6819.49706544334, 6829.81917219631, 6840.04830175026, 6850.18646570771, 6860.23560335127, 6870.19758495911, 6880.07421495093, 6889.86723487356, 6899.57832623505, 6909.20911319526, 6918.76116512077, 6928.2359990113, 6937.63508180467, 6946.95983256654, 6956.21162457125, 6965.39178727937, 6974.50160821762, 6983.54233476606, 6992.51517585762, 7001.42130359452, 7010.26185478586, 7019.03793241062, 7027.75060700985, 7036.40091801184, 7044.98987499363, 7053.5184588823, 7061.987623099, 7070.39829464883, 7078.75137515927, 7087.04774186974, 7095.28824857502, 7103.47372652462, 7111.60498528053, 7119.6828135354, 7127.7079798932, 7135.68123361421, 7143.60330532614, 7149.03377676516, 7150.60519864653, 7151.47490770318, 7159.29673611448, 7167.06946924362, 7174.79376968062, 7182.47028448767, 7190.09964574004, 7197.68247104339, 7205.21936402852, 7212.71091482481, 7220.15770051333, 7227.56028556059, 7234.91922223393, 7242.23505099943, 7249.50830090311, 7256.73948993633, 7263.92912538609, 7271.0777041709, 7278.18571316309, 7285.25362949795, ...(+4235 chars)] J/(K*kg)  Dij=[20; 18; 70; 25] mm^2/s  Ru=8.3144598 J/(K*mol)  R=[296.80220443872; 259.836700688776; 4124.48291465762; 461.523115726061] J/(K*kg)  p_amb=101325 Pa  T_amb=293.15 K  p_min=1 kPa  T_min=225 K  can_cond=[0; 0; 0; 1]
      settings: InternalSimscapePortConfiguration="{\"Bottom\":[],\"Left\":[{\"id\":\"A\",\"label\":\"A\",\"type\":\"FuelCell.FuelCell\"}],\"Right\":[],\"Top\":[]}"
  Heat Dissipation : Subsystem
      settings: PortSchema="{\"entries\":[{\"content\":{\"sides\":[{\"content\":{\"connectorIds\":[]},\"type\":\"ConnectorPlacement.EquallySpacedRectSide\",\"uuid\":\"40b2385a-b20e-464f-8016-3228e4acac4a\"},{\"content\":{\"connectorIds\":[],\"side\":\"RIGHT\"},\"type\":\"ConnectorPlacement.EquallySpacedRectSide\",\"uuid\":\"0e95dc4b-d2da-4ab6-a6e9-e2cb275776ce\"},{\"content\":{\"connectorIds\":[\"LConn1\"],\"side\":\"TOP\"},\"type\":\"ConnectorPlacement.EquallySpacedRectSide\",\"uuid\":\"0f5995c7-26f6-433d-889b-dea78bcd2b2a\"},{\"content\":{\"connectorIds\":[\"RConn1\"],\"side\":\"BOTTOM\"},\"type\":\"ConnectorPlacement.EquallySpacedRectSide\",\"uuid\":\"a2ee1c19-f9e9-4dbd-a9ff-92feea387e85\"}]},\"type\":\"ConnectorPlacement.EquallySpacedConnector\",\"uuid\":\"721753ea-9ada-4c74-8c6f-50b905d96904\"}],\"packageUris\":[\"http://schema.mathworks.com/mf0/Connector/R2020b\"],\"version\":\"1.0\"}"
  Hydrogen Source : Subsystem  Tag=PublishSubsystem
      mask Display:
      | plot(0, 0)
      | plot(100, 100)
      | 
      | n = 20;
      | r = 20;
      | x1 = 15;
      | x2 = 65;
      | y1 = 5;
      | y2 = 85;
      | 
      | plot([x1 x1], [y1+r y2-r])
      | plot([x1+r x2-r], [y2 y2])
      | plot([x2 x2], [y2-r y1+r])
      | plot([x2-r x1+r], [y1 y1])
      | 
      | plot(cos(linspace(pi/2, pi, n))*r + x1+r, sin(linspace(pi/2, pi, n))*r + y2-r)
      | plot(cos(linspace(0, pi/2, n))*r + x2-r, sin(linspace(0, pi/2, n))*r + y2-r)
      | plot(cos(linspace(3*pi/2, 2*pi, n))*r + x2-r, sin(linspace(3*pi/2, 2*pi, n))*r + y1+r)
      | plot(cos(linspace(pi, 3*pi/2, n))*r + x1+r, sin(linspace(pi, 3*pi/2, n))*r + y1+r)
      | 
      | plot([-5 -5 5 5] + (x1+x2)/2, [0 5 5 0] + y2)
  MEA Thermal Mass : fl_lib/Thermal/Thermal Elements/Thermal Mass  mass_type=foundation.enum.constant_variable.constant  mass=stack_mea_rho * stack_area*1e-4 * (stack_t_membrane + 2*stack_t_gdl)*1e-6 * stack_num_cells kg  sp_heat=stack_mea_cp J/kg/K  mass_min=1e-6 kg  num_ports=foundation.enum.numPorts2.one  m_specify=off  m_priority=High  m=1 kg  m_nominal_specify=off  m_nominal_value=1  m_nominal_unit=kg  T_specify=on  T_priority=High  T=env_T degC  T_nominal_specify=off  T_nominal_value=1  T_nominal_unit=K  Q_specify=off  Q_priority=None  Q=0 W  Q_nominal_specify=off  Q_nominal_value=1  Q_nominal_unit=W
  Measurements : Subsystem
  Membrane Electrode Assembly : FuelCell_lib/elements/Membrane Electrode Assembly  N_cell=stack_num_cells  area_cell=stack_area cm^2  t_membrane=stack_t_membrane um  rtype=FuelCell.enum.ResistanceModel.Tabulated1D  RH_TLU=[0, .1, .2, .3, .4, .5, .6, .7, .8, .9, 1]  conductivity_TLU_1D=[0, .017, .035, .055, .081, .11, .15, .21, .27, .35, .45] S/cm  T_scale=1268 K  T_cond=353.15 K  T_TLU=[303.15, 353.15, 393.15] K  conductivity_TLU_2D=[0, .0093, .019, .031, .045, .063, .086, .11, .15, .2, .25; 0, .017, .035, .055, .081, .11, .15, .21, .27, .35, .45; 0, .024, .05, .08, .12, .16, .22, .3, .39, .51, .65] S/cm  io=stack_io A/cm^2  iL=stack_iL A/cm^2  alpha=stack_alpha  rho_membrane=2000 kg/m^3  M_membrane=1.1 kg/mol  D_N2=1e-5 cm^2/s  Icell_specify=off  Icell_priority=None  Icell=0 A  Icell_nominal_specify=off  Icell_nominal_value=1  Icell_nominal_unit=A  HeatRxn_specify=off  HeatRxn_priority=None  HeatRxn=0 W  HeatRxn_nominal_specify=off  HeatRxn_nominal_value=1  HeatRxn_nominal_unit=W  T_stack_specify=off  T_stack_priority=None  T_stack=353.15 K  T_stack_nominal_specify=off  T_stack_nominal_value=1  T_stack_nominal_unit=K
      settings: InternalSimscapePortConfiguration="{\"Bottom\":[{\"id\":\"H\",\"label\":\"H\",\"type\":\"foundation.thermal.thermal\"}],\"Left\":[{\"id\":\"A\",\"label\":\"A\",\"type\":\"FuelCell.FuelCell\"},{\"id\":\"mdot_an\",\"label\":\"Ma\",\"type\":\"output\"},{\"id\":\"T_an\",\"label\":\"Ta\",\"type\":\"output\"},{\"id\":\"x_i_anode\",\"label\":\"xia\",\"type\":\"input\"}],\"Right\":[{\"id\":\"C\",\"label\":\"C\",\"type\":\"FuelCell.FuelCell\"},{\"id\":\"mdot_ca\",\"label\":\"Mc\",\"type\":\"output\"},{\"id\":\"T_ca\",\"label\":\"Tc\",\"type\":\"output\"},{\"id\":\"x_i_cathode\",\"label\":\"xic\",\"type\":\"input\"}],\"Top\":[{\"id\":\"n\",\"label\":\"-\",\"type\":\"foundation.electrical.electrical\"},{\"id\":\"p\",\"label\":\"+\",\"type\":\"foundation.electrical.electrical\"}]}"
  N2 Tracking : Scope  NumInputPorts=2
      settings: Title=Anode Nitrogen Molar Fraction and Purge Valve Activation  ActiveDisplayYMinimum=-0.125  ActiveDisplayYMaximum=1.125
  Oxygen Source : Subsystem  Tag=PublishSubsystem
      mask Display:
      | plot(0, 0)
      | plot(100, 100)
      | 
      | n = 80;
      | r1 = 15;
      | r2 = 30;
      | 
      | plot(cos(linspace(0, 2*pi, n))*r1 + 65, sin(linspace(0, 2*pi, n))*r1 + 50)
      | plot(cos(linspace(0, 2*pi, n))*r2 + 65, sin(linspace(0, 2*pi, n))*r2 + 50)
      | 
      | plot([65 30 30 42], [80 80 70 70])
  Performance : Scope  NumInputPorts=4
      settings: Title=Current (A)  ActiveDisplayYMinimum=-30.6721  ActiveDisplayYMaximum=276.0489
  Recirculation : Subsystem  Tag=PublishSubsystem
      settings: PortSchema="{\"entries\":[{\"content\":{\"sides\":[{\"content\":{\"connectorIds\":[\"LConn1\"]},\"type\":\"ConnectorPlacement.EquallySpacedRectSide\",\"uuid\":\"a905d28b-4136-4e4b-b56f-ff4ef454860e\"},{\"content\":{\"connectorIds\":[\"RConn1\"],\"side\":\"RIGHT\"},\"type\":\"ConnectorPlacement.EquallySpacedRectSide\",\"uuid\":\"7d453241-460d-4f71-8108-f868ae96b726\"},{\"content\":{\"connectorIds\":[],\"side\":\"TOP\"},\"type\":\"ConnectorPlacement.EquallySpacedRectSide\",\"uuid\":\"5de5a8e7-eaa9-43ea-9e3e-e109b24be5c4\"},{\"content\":{\"connectorIds\":[\"RConn2\"],\"side\":\"BOTTOM\"},\"type\":\"ConnectorPlacement.EquallySpacedRectSide\",\"uuid\":\"9c44ad98-d3d2-40d8-a226-ad16e20687d9\"}]},\"type\":\"ConnectorPlacement.EquallySpacedConnector\",\"uuid\":\"be431bc9-ad83-41b5-a4a3-7fe11e97fedb\"}],\"packageUris\":[\"http://schema.mathworks.com/mf0/Connector/R2020b\"],\"version\":\"1.0\"}"
  Solver Configuration : nesl_utility/Solver Configuration  PhysicalDomain=network_engine_domain  SubClassName=solver  LeftPortType=input  RightPortType=generic  Tones=[]  Harmonics=[]  SimulateNoise=off  Profile=off  UseLocalSampling=off  EnableSwitchedLinearOptims=on  FrequencyDomain=off  UseCCode=off  RelTol=0.001  AbsTol=1e-06  MinStep=1e-09  ToWorkspace=off  RevertToSquareIcSolve=off  NumHomotopyIterations=100  PhasorMode=off  PhasorModeNumHarmonics=1  ConsistencySolver=NEWTON_XTOL_AFTER_FTOL  IndexReductionMethod=DerivativeReplacement  DoDC=off  ResidualTolerance=1e-09  ConsistencyTolSource=GLOBAL  ConsistencyAbsTol=0.001  ConsistencyRelTol=0.001  ConsistencyTolFactor=0.001  UseLocalSolver=off  LocalSolverChoice=NE_BACKWARD_EULER_ADVANCER  ResolveIndetEquations=on  FunctionEvalNumThread=1  LocalSolverSampleTime=0.001  DoFixedCost=off  MaxNonlinIter=3  MaxModeIter=2  ComputeImpulses=off  ImpulseIterations=2  LinearAlgebra=auto  LinearAlgebraNumThread=0  EquationFormulation=NE_TIME_EF  DelaysMemoryBudget=1024  AutomaticFiltering=on  FilteringTimeConstant=0.001  PartitionStorageMethod=AS_NEEDED  PartitionMemoryBudget=1024  PartitionMethod=ROBUST  MultibodyUseLocalSolver=off  MultibodyLocalSolverChoice=ODE1  MultibodyLocalSolverSampleTime=0.001
  Subsystem : Subsystem
  wires:
  Measurements/1(i) -> Performance/1
  Measurements/2(v) -> Performance/2
  Measurements/3(P) -> Performance/3
  Measurements/4(T) -> Performance/4
  Subsystem/1(N2) -> N2 Tracking/1  "yN2"
  Subsystem/2(Purge) -> N2 Tracking/2  "Activated Valve"
  connections:
  Anode Gas Channels/RConn1 -- Membrane Electrode Assembly/LConn1
  Anode Humidifier/LConn1 -- Recirculation/RConn1
  Heat Dissipation/RConn1 -- Solver Configuration/RConn1 -- MEA Thermal Mass/LConn1 -- Cooling System/RConn1 -- Convective Heat Transfer1/RConn1 -- Convective Heat Transfer2/RConn1
  Recirculation/LConn1 -- Hydrogen Source/RConn1
  Recirculation/RConn2 -- Gas Mixture Properties/LConn1 -- Anode Exhaust/LConn1 -- Anode Gas Channels/LConn2
  Anode Gas Channels/LConn3 -- Membrane Electrode Assembly/LConn4
  Membrane Electrode Assembly/RConn5 -- Heat Dissipation/LConn1
  Anode Gas Channels/RConn3 -- Membrane Electrode Assembly/LConn3
  Anode Gas Channels/RConn2 -- Membrane Electrode Assembly/LConn2
  Cathode Gas Channels/LConn2 -- Cathode Exhaust/LConn1
  Cathode Gas Channels/LConn1 -- Cathode Humidifier/LConn1
  Cathode Humidifier/RConn1 -- Oxygen Source/LConn1
  Anode Humidifier/RConn1 -- Anode Gas Channels/LConn1
  Electrical Load/RConn1 -- Membrane Electrode Assembly/LConn5
  Electrical Load/RConn2 -- Membrane Electrode Assembly/LConn6
  Convective Heat Transfer2/LConn1 -- Anode Gas Channels/RConn4
  Convective Heat Transfer1/LConn1 -- Cathode Gas Channels/RConn4
  Membrane Electrode Assembly/RConn1 -- Cathode Gas Channels/RConn1
  Membrane Electrode Assembly/RConn2 -- Cathode Gas Channels/RConn2
  Membrane Electrode Assembly/RConn3 -- Cathode Gas Channels/RConn3
  Membrane Electrode Assembly/RConn4 -- Cathode Gas Channels/LConn3
